simulink model "battery_model_closed_loop_simscape"  (R2016a)
settings: Solver=VariableStepAuto  StartTime=0.0  StopTime=6000  RelTol=1e-3
values from neighbouring files (symbols this model uses):
  C1 = tau1/R1    (= 240000)    [battery_and_controller_simscape_parameters.m]
  Cc = 1/(Q*wn*Rc)    [battery_and_controller_simscape_parameters.m]
  Ch = tauh/Rh    (= 40000)    [battery_and_controller_simscape_parameters.m]
  Cnom = 10    [battery_and_controller_simscape_parameters.m]
  Crate = 1.5*Mp*Cnom    (= 45)    [battery_and_controller_simscape_parameters.m]
  Gc0 = Gcwc*abs((1/wcp)*(i*wc)^2+(i*wc)+1)    [battery_and_controller_simscape_parameters.m]
  Lc = 1/(wn^2*Cc)    [battery_and_controller_simscape_parameters.m]
  Mp = 3    [battery_and_controller_simscape_parameters.m]
  Ns = 100    [battery_and_controller_simscape_parameters.m]
  R1 = 1e-3    (= 0.001)    [battery_and_controller_simscape_parameters.m]
  Rc = 5e3    (= 5000)    [battery_and_controller_simscape_parameters.m]
  Rs = Rp    (= 0.005)    [battery_and_controller_simscape_parameters.m]
  SOC_1 = 0.8    [battery_and_controller_simscape_parameters.m]
undefined symbols (not defined in the file or in its folder): V_soc
libraries: powerlib x49
settings Model: Creator=Gorkem  LastModifiedBy=Gorkem

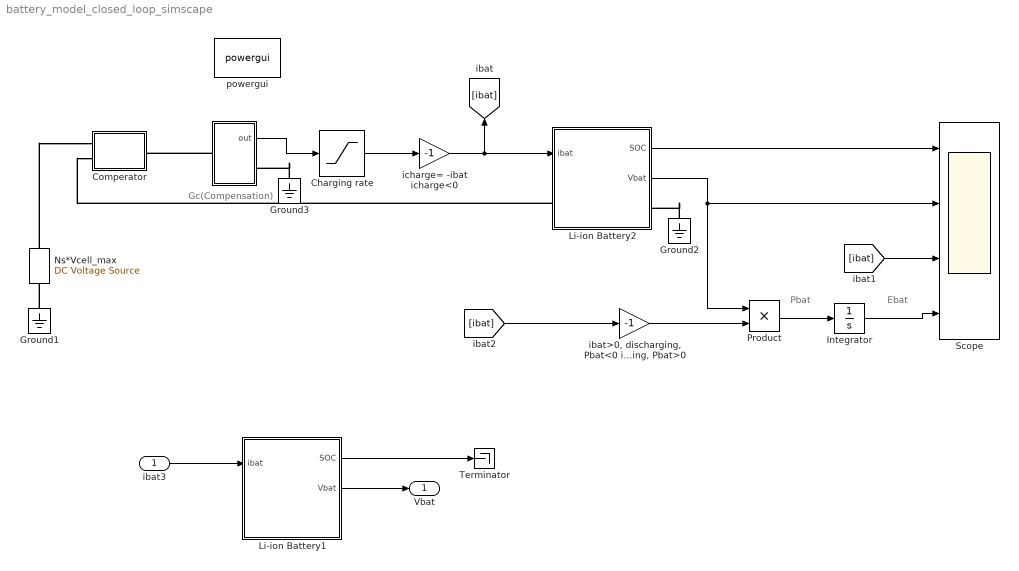
== system battery_model_closed_loop_simscape ==
  note: Gc(Compensation)
  note: Ebat
  note: Pbat
  ibat3 : Inport
  "  " : Subsystem
  Charging rate : Saturate  UpperLimit=Crate  LowerLimit=0
  Comperator : Subsystem
  Ground1 : powerlib/Elements/Ground  LConnTagsString=a
  Ground2 : powerlib/Elements/Ground  LConnTagsString=a
  Ground3 : powerlib/Elements/Ground  LConnTagsString=a
  Integrator : Integrator
  Li-ion Battery1 : Subsystem
  Li-ion Battery2 : Subsystem
  Ns*Vcell_max : powerlib/Electrical Sources/DC Voltage Source  Amplitude=3.7*Ns  Measurements=None
  Product : Product
  Scope : Scope  NumInputPorts=4
  Terminator : Terminator
  "ibat>0, discharging, Pbat<0 ibat<0, charging, Pbat>0" : Gain  Gain=-1
  icharge= -ibat icharge<0 : Gain  Gain=-1
  powergui : powerlib/powergui  Priority=1  SimulationMode=Continuous  SolverType=Tustin/Backward Euler (TBE)  SampleTime=50e-6  frequency=60  SPID=off  DisableSnubberDevices=off  DisableRonSwitches=off  DisableVfSwitches=off  SwTol=0  DisplayEquations=off  Interpol=off  ExternalGateDelay=off  methode=off  Ts=10  FunctionMessages=off  echomessages=off  HookPort=off  EnableUseOfTLC=off  x0status=blocks  frequencyindice=0  Pbase=100e6  ErrMax=1e-4  Iterations=50  UnitsV=kV  UnitsW=MW  buscounter=0  RestoreLinks=warning  ResistiveCurrentMeasurement=off  Frange=[0:2:500]  Ylog=off  Xlog=on  ShowGrid=off  save=off  variable=ZData  structure=0  ZoomFFT=off  StartTime=0.0  cycles=1  DisplayStyle=1  fundamental=60  FreqAxis=off  MaxFrequency=1000  frequencyindicesteady=1  RmsSteady=1  display=off
  Vbat : Outport
  wires:
  icharge= -ibat icharge<0/1 -> [ibat], Li-ion Battery2/1(ibat)
  Product/1 -> Integrator/1
  "ibat>0, discharging, Pbat<0 ibat<0, charging, Pbat>0"/1 -> Product/2
  Integrator/1 -> Scope/4
  Charging rate/1 -> icharge= -ibat icharge<0/1
  Li-ion Battery2/2(Vbat) -> Product/1, Scope/2
  Li-ion Battery2/1(SOC) -> Scope/1
  "  "/1("out ") -> Charging rate/1
  [ibat] -> "ibat>0, discharging, Pbat<0 ibat<0, charging, Pbat>0"/1
  [ibat] -> Scope/3
  ibat3/1 -> Li-ion Battery1/1(ibat)
  Li-ion Battery1/2(Vbat) -> Vbat/1
  Li-ion Battery1/1(SOC) -> Terminator/1
  connections:
  Ground1/LConn1 -- Ns*Vcell_max/LConn1
  Ground2/LConn1 -- Li-ion Battery2/RConn1
  Li-ion Battery2/LConn1 -- Comperator/LConn2
  Ns*Vcell_max/RConn1 -- Comperator/LConn1
  "  "/LConn1 -- Comperator/RConn1
  Ground3/LConn1 -- "  "/RConn1

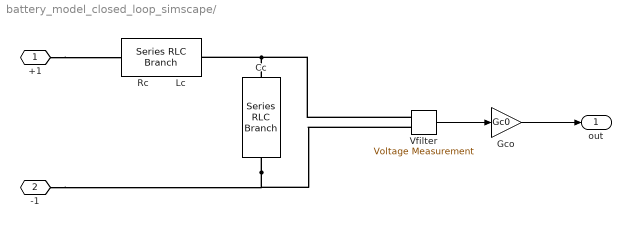
== system battery_model_closed_loop_simscape/   ==
  Cc : powerlib/Elements/Series RLC Branch  LConnTagsString=__new0  RConnTagsString=__new0  BranchType=C  Resistance=Rc  Inductance=Lc  SetiL0=off  InitialCurrent=0  Capacitance=Cc  Setx0=off  InitialVoltage=0  Measurements=None
  Gco : Gain  Gain=Gc0
  Rc         Lc : powerlib/Elements/Series RLC Branch  LConnTagsString=__new0  RConnTagsString=__new0  BranchType=RL  Resistance=Rc  Inductance=Lc  SetiL0=off  InitialCurrent=0  Capacitance=1e-6  Setx0=off  InitialVoltage=0  Measurements=None
  "Vfilter " : powerlib/Measurements/Voltage Measurement  PhasorSimulation=off  OutputType=Complex  PSBequivalent=0
  +1 : PMIOPort  Port=1  Side=Left
  -1 : PMIOPort  Port=2  Side=Right
  "out " : Outport
  wires:
  "Vfilter "/1 -> Gco/1
  Gco/1 -> "out "/1
  connections:
  +1/RConn1 -- Rc         Lc/LConn1
  Cc/LConn1 -- "Vfilter "/LConn1 -- Rc         Lc/RConn1
  Cc/RConn1 -- "Vfilter "/LConn2 -- -1/RConn1

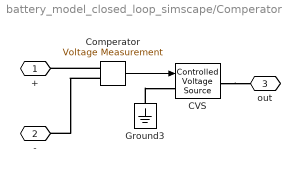
== system battery_model_closed_loop_simscape/Comperator ==
  CVS : powerlib/Electrical Sources/Controlled Voltage Source  Initialize=on  Source_Type=AC  Amplitude=0  Phase=0  Frequency=0  Measurements=None
  Comperator : powerlib/Measurements/Voltage Measurement  PhasorSimulation=off  OutputType=Complex  PSBequivalent=0
  Ground3 : powerlib/Elements/Ground  LConnTagsString=a
  + : PMIOPort  Port=1  Side=Left
  - : PMIOPort  Port=2  Side=Left
  out : PMIOPort  Port=3  Side=Right
  wires:
  Comperator/1 -> CVS/1
  connections:
  Ground3/LConn1 -- CVS/LConn1
  CVS/RConn1 -- out/RConn1
  Comperator/LConn2 -- -/RConn1
  Comperator/LConn1 -- +/RConn1

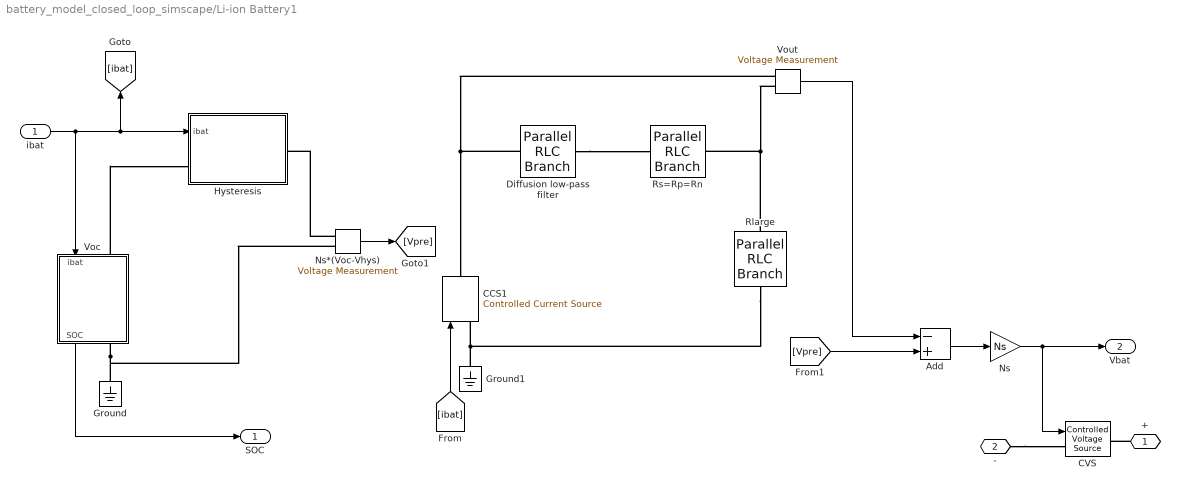
== system battery_model_closed_loop_simscape/Li-ion Battery1 ==
  ibat : Inport
  Add : Sum  Inputs=-+
  CCS1 : powerlib/Electrical Sources/Controlled Current Source  Initialize=off  Source_Type=AC  Amplitude=0  Phase=0  Frequency=0  Measurements=Current
  CVS : powerlib/Electrical Sources/Controlled Voltage Source  Initialize=on  Source_Type=AC  Amplitude=0  Phase=0  Frequency=0  Measurements=None
  Diffusion low-pass filter : powerlib/Elements/Parallel RLC Branch  LConnTagsString=a  RConnTagsString=__new0  BranchType=RC  Resistance=R1/Mp  Inductance=1e-3  SetiL0=off  InitialCurrent=0  Capacitance=C1*Mp  Setx0=off  InitialVoltage=0  Measurements=None
  Ground : powerlib/Elements/Ground  LConnTagsString=a
  Ground1 : powerlib/Elements/Ground  LConnTagsString=a
  Hysteresis : Subsystem
  Ns : Gain  Gain=Ns
  Ns*(Voc-Vhys) : powerlib/Measurements/Voltage Measurement  PhasorSimulation=off  OutputType=Complex  PSBequivalent=0
  Rlarge : powerlib/Elements/Parallel RLC Branch  LConnTagsString=a  RConnTagsString=__new0  BranchType=R  Resistance=1e15  Inductance=1e-3  SetiL0=off  InitialCurrent=0  Capacitance=C1*(Mp/Ns)  Setx0=off  InitialVoltage=0  Measurements=None
  Rs=Rp=Rn : powerlib/Elements/Parallel RLC Branch  LConnTagsString=a  RConnTagsString=__new0  BranchType=R  Resistance=Rs/Mp  Inductance=1e-3  SetiL0=off  InitialCurrent=0  Capacitance=C1*(Mp/Ns)  Setx0=off  InitialVoltage=0  Measurements=None
  Voc : Subsystem
  Vout : powerlib/Measurements/Voltage Measurement  PhasorSimulation=off  OutputType=Complex  PSBequivalent=0
  + : PMIOPort  Port=1  Side=Left
  - : PMIOPort  Port=2  Side=Right
  SOC : Outport
  Vbat : Outport  Port=2
  wires:
  Voc/1(SOC) -> SOC/1
  ibat/1 -> Voc/1(ibat), [ibat], Hysteresis/1(ibat)
  [ibat] -> CCS1/1
  Vout/1 -> Add/1
  Ns*(Voc-Vhys)/1 -> [Vpre]
  [Vpre] -> Add/2
  Add/1 -> Ns/1
  Ns/1 -> CVS/1, Vbat/1
  connections:
  Voc/LConn1 -- Hysteresis/LConn1
  Voc/RConn1 -- Ground/LConn1 -- Ns*(Voc-Vhys)/LConn2
  Diffusion low-pass filter/LConn1 -- Vout/LConn1 -- CCS1/RConn1
  Ground1/LConn1 -- CCS1/LConn1 -- Rlarge/RConn1
  Diffusion low-pass filter/RConn1 -- Rs=Rp=Rn/LConn1
  Vout/LConn2 -- Rlarge/LConn1 -- Rs=Rp=Rn/RConn1
  Ns*(Voc-Vhys)/LConn1 -- Hysteresis/RConn1
  +/RConn1 -- CVS/RConn1
  -/RConn1 -- CVS/LConn1

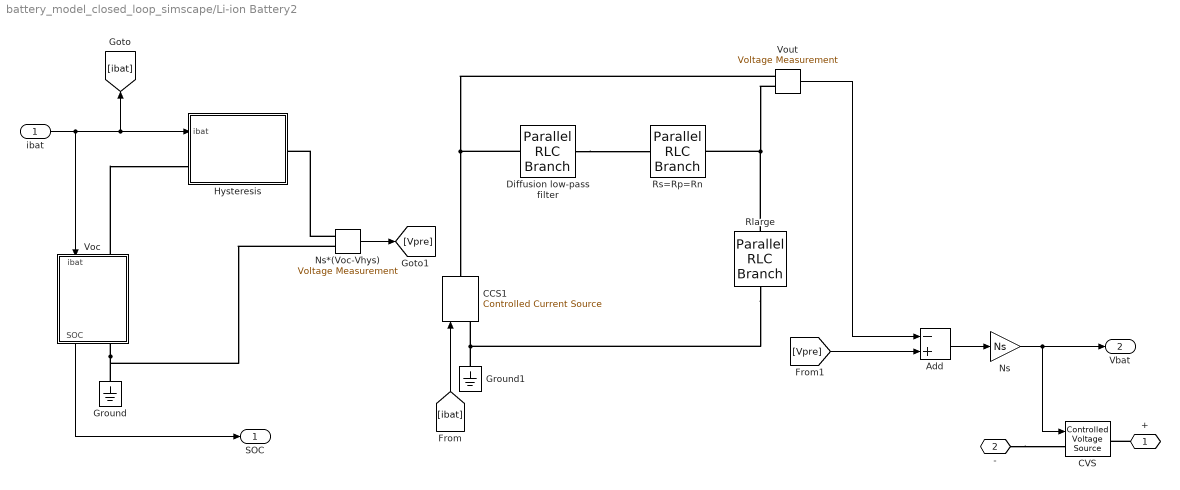
== system battery_model_closed_loop_simscape/Li-ion Battery2 ==
  ibat : Inport
  Add : Sum  Inputs=-+
  CCS1 : powerlib/Electrical Sources/Controlled Current Source  Initialize=off  Source_Type=AC  Amplitude=0  Phase=0  Frequency=0  Measurements=Current
  CVS : powerlib/Electrical Sources/Controlled Voltage Source  Initialize=on  Source_Type=AC  Amplitude=0  Phase=0  Frequency=0  Measurements=None
  Diffusion low-pass filter : powerlib/Elements/Parallel RLC Branch  LConnTagsString=a  RConnTagsString=__new0  BranchType=RC  Resistance=R1/Mp  Inductance=1e-3  SetiL0=off  InitialCurrent=0  Capacitance=C1*Mp  Setx0=off  InitialVoltage=0  Measurements=None
  Ground : powerlib/Elements/Ground  LConnTagsString=a
  Ground1 : powerlib/Elements/Ground  LConnTagsString=a
  Hysteresis : Subsystem
  Ns : Gain  Gain=Ns
  Ns*(Voc-Vhys) : powerlib/Measurements/Voltage Measurement  PhasorSimulation=off  OutputType=Complex  PSBequivalent=0
  Rlarge : powerlib/Elements/Parallel RLC Branch  LConnTagsString=a  RConnTagsString=__new0  BranchType=R  Resistance=1e15  Inductance=1e-3  SetiL0=off  InitialCurrent=0  Capacitance=C1*(Mp/Ns)  Setx0=off  InitialVoltage=0  Measurements=None
  Rs=Rp=Rn : powerlib/Elements/Parallel RLC Branch  LConnTagsString=a  RConnTagsString=__new0  BranchType=R  Resistance=Rs/Mp  Inductance=1e-3  SetiL0=off  InitialCurrent=0  Capacitance=C1*(Mp/Ns)  Setx0=off  InitialVoltage=0  Measurements=None
  Voc : Subsystem
  Vout : powerlib/Measurements/Voltage Measurement  PhasorSimulation=off  OutputType=Complex  PSBequivalent=0
  + : PMIOPort  Port=1  Side=Left
  - : PMIOPort  Port=2  Side=Right
  SOC : Outport
  Vbat : Outport  Port=2
  wires:
  Voc/1(SOC) -> SOC/1
  ibat/1 -> Voc/1(ibat), [ibat], Hysteresis/1(ibat)
  [ibat] -> CCS1/1
  Vout/1 -> Add/1
  Ns*(Voc-Vhys)/1 -> [Vpre]
  [Vpre] -> Add/2
  Add/1 -> Ns/1
  Ns/1 -> CVS/1, Vbat/1
  connections:
  Voc/LConn1 -- Hysteresis/LConn1
  Voc/RConn1 -- Ground/LConn1 -- Ns*(Voc-Vhys)/LConn2
  Diffusion low-pass filter/LConn1 -- Vout/LConn1 -- CCS1/RConn1
  Ground1/LConn1 -- CCS1/LConn1 -- Rlarge/RConn1
  Diffusion low-pass filter/RConn1 -- Rs=Rp=Rn/LConn1
  Vout/LConn2 -- Rlarge/LConn1 -- Rs=Rp=Rn/RConn1
  Ns*(Voc-Vhys)/LConn1 -- Hysteresis/RConn1
  +/RConn1 -- CVS/RConn1
  -/RConn1 -- CVS/LConn1

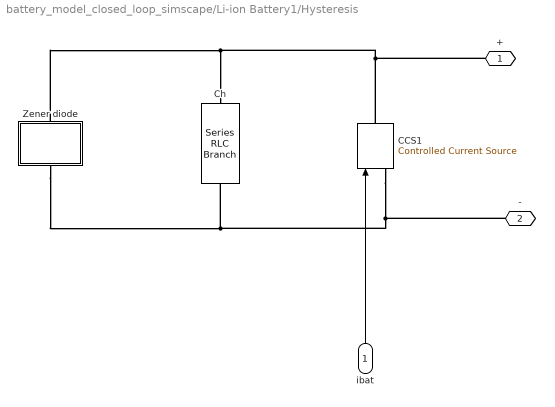
== system battery_model_closed_loop_simscape/Li-ion Battery1/Hysteresis ==
  ibat : Inport
  CCS1 : powerlib/Electrical Sources/Controlled Current Source  Initialize=off  Source_Type=AC  Amplitude=0  Phase=0  Frequency=0  Measurements=Current
  Ch : powerlib/Elements/Series RLC Branch  LConnTagsString=__new0  RConnTagsString=__new0  BranchType=C  Resistance=1  Inductance=1e-3  SetiL0=off  InitialCurrent=0  Capacitance=(Mp/Ns)*Ch  Setx0=off  InitialVoltage=0  Measurements=None
  Zener diode : Subsystem
  + : PMIOPort  Port=1  Side=Left
  - : PMIOPort  Port=2  Side=Right
  wires:
  ibat/1 -> CCS1/1
  connections:
  Zener diode/LConn1 -- Ch/LConn1 -- CCS1/RConn1 -- +/RConn1
  Zener diode/RConn1 -- Ch/RConn1 -- -/RConn1 -- CCS1/LConn1

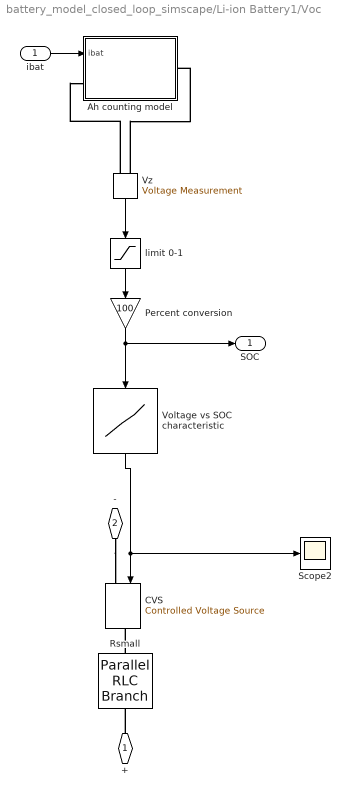
== system battery_model_closed_loop_simscape/Li-ion Battery1/Voc ==
  ibat : Inport
  Ah counting model : Subsystem
  CVS : powerlib/Electrical Sources/Controlled Voltage Source  Initialize=off  Source_Type=AC  Amplitude=0  Phase=0  Frequency=0  Measurements=Voltage
  Percent conversion : Gain  Gain=100
  Rsmall : powerlib/Elements/Parallel RLC Branch  LConnTagsString=a  RConnTagsString=__new0  BranchType=R  Resistance=1e-15  Inductance=1e-3  SetiL0=off  InitialCurrent=0  Capacitance=C1*(Mp/Ns)  Setx0=off  InitialVoltage=0  Measurements=None
  Scope2 : Scope
  Voltage vs SOC characteristic : Lookup_n-D  NumberOfTableDimensions=1  BreakpointsForDimension1=[0:9900]/100  Table=V_soc  InternalRulePriority=Speed  RndMeth=Simplest  InputSameDT=on
  Vz : powerlib/Measurements/Voltage Measurement  PhasorSimulation=off  OutputType=Complex  PSBequivalent=0
  limit 0-1 : Saturate  UpperLimit=SOC_1  LowerLimit=0
  + : PMIOPort  Port=1  Side=Left
  - : PMIOPort  Port=2  Side=Right
  SOC : Outport
  wires:
  Percent conversion/1 -> SOC/1, Voltage vs SOC characteristic/1
  Voltage vs SOC characteristic/1 -> Scope2/1, CVS/1
  Vz/1 -> limit 0-1/1
  limit 0-1/1 -> Percent conversion/1
  ibat/1 -> Ah counting model/1(ibat)
  connections:
  Vz/LConn2 -- Ah counting model/RConn1
  +/RConn1 -- Rsmall/RConn1
  Vz/LConn1 -- Ah counting model/LConn1
  -/RConn1 -- CVS/LConn1
  Rsmall/LConn1 -- CVS/RConn1

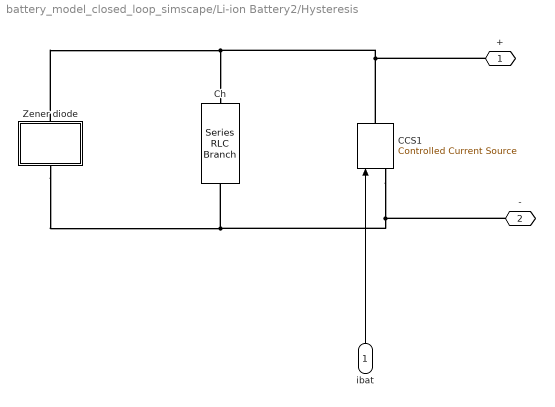
== system battery_model_closed_loop_simscape/Li-ion Battery2/Hysteresis ==
  ibat : Inport
  CCS1 : powerlib/Electrical Sources/Controlled Current Source  Initialize=off  Source_Type=AC  Amplitude=0  Phase=0  Frequency=0  Measurements=Current
  Ch : powerlib/Elements/Series RLC Branch  LConnTagsString=__new0  RConnTagsString=__new0  BranchType=C  Resistance=1  Inductance=1e-3  SetiL0=off  InitialCurrent=0  Capacitance=(Mp/Ns)*Ch  Setx0=off  InitialVoltage=0  Measurements=None
  Zener diode : Subsystem
  + : PMIOPort  Port=1  Side=Left
  - : PMIOPort  Port=2  Side=Right
  wires:
  ibat/1 -> CCS1/1
  connections:
  Zener diode/LConn1 -- Ch/LConn1 -- CCS1/RConn1 -- +/RConn1
  Zener diode/RConn1 -- Ch/RConn1 -- -/RConn1 -- CCS1/LConn1

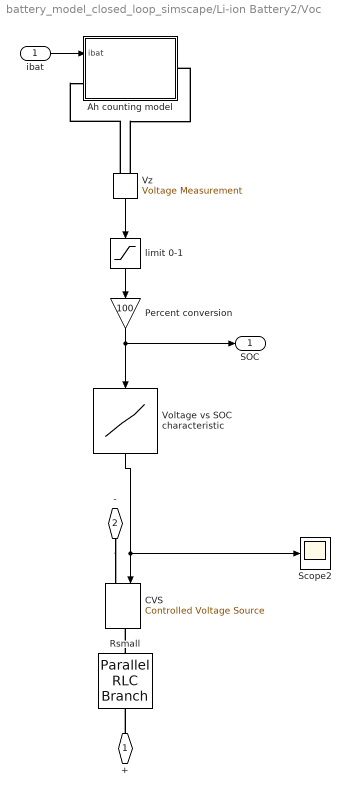
== system battery_model_closed_loop_simscape/Li-ion Battery2/Voc ==
  ibat : Inport
  Ah counting model : Subsystem
  CVS : powerlib/Electrical Sources/Controlled Voltage Source  Initialize=off  Source_Type=AC  Amplitude=0  Phase=0  Frequency=0  Measurements=Voltage
  Percent conversion : Gain  Gain=100
  Rsmall : powerlib/Elements/Parallel RLC Branch  LConnTagsString=a  RConnTagsString=__new0  BranchType=R  Resistance=1e-15  Inductance=1e-3  SetiL0=off  InitialCurrent=0  Capacitance=C1*(Mp/Ns)  Setx0=off  InitialVoltage=0  Measurements=None
  Scope2 : Scope
  Voltage vs SOC characteristic : Lookup_n-D  NumberOfTableDimensions=1  BreakpointsForDimension1=[0:9900]/100  Table=V_soc  InternalRulePriority=Speed  RndMeth=Simplest  InputSameDT=on
  Vz : powerlib/Measurements/Voltage Measurement  PhasorSimulation=off  OutputType=Complex  PSBequivalent=0
  limit 0-1 : Saturate  UpperLimit=SOC_1  LowerLimit=0
  + : PMIOPort  Port=1  Side=Left
  - : PMIOPort  Port=2  Side=Right
  SOC : Outport
  wires:
  Percent conversion/1 -> SOC/1, Voltage vs SOC characteristic/1
  Voltage vs SOC characteristic/1 -> Scope2/1, CVS/1
  Vz/1 -> limit 0-1/1
  limit 0-1/1 -> Percent conversion/1
  ibat/1 -> Ah counting model/1(ibat)
  connections:
  Vz/LConn2 -- Ah counting model/RConn1
  +/RConn1 -- Rsmall/RConn1
  Vz/LConn1 -- Ah counting model/LConn1
  -/RConn1 -- CVS/LConn1
  Rsmall/LConn1 -- CVS/RConn1

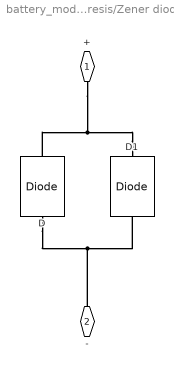
== system battery_model_closed_loop_simscape/Li-ion Battery1/Hysteresis/Zener diode ==
  D : powerlib/Power Electronics/Diode  Ron=0.001  Lon=0  Vf=Vm  IC=0  UseSnubber=off  Rs=inf  Cs=0  Measurements=off
  D1 : powerlib/Power Electronics/Diode  Ron=0.001  Lon=0  Vf=Vm  IC=0  UseSnubber=off  Rs=inf  Cs=0  Measurements=off
  + : PMIOPort  Port=1  Side=Left
  - : PMIOPort  Port=2  Side=Right
  connections:
  D1/LConn1 -- D/RConn1 -- +/RConn1
  D1/RConn1 -- D/LConn1 -- -/RConn1

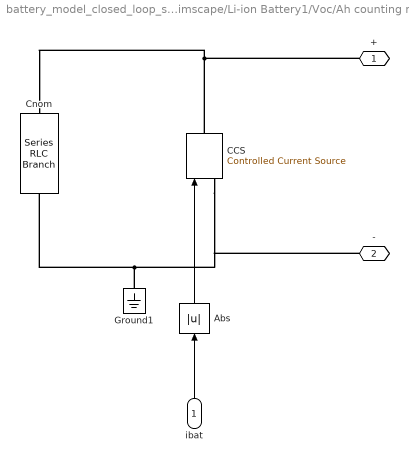
== system battery_model_closed_loop_simscape/Li-ion Battery1/Voc/Ah counting model ==
  ibat : Inport
  Abs : Abs
  CCS : powerlib/Electrical Sources/Controlled Current Source  Initialize=off  Source_Type=AC  Amplitude=0  Phase=0  Frequency=0  Measurements=Current
  Cnom : powerlib/Elements/Series RLC Branch  LConnTagsString=__new0  RConnTagsString=__new0  BranchType=C  Resistance=1  Inductance=1e-3  SetiL0=off  InitialCurrent=0  Capacitance=Cnom*Mp*3600  Setx0=on  InitialVoltage=SOC_0  Measurements=None
  Ground1 : powerlib/Elements/Ground  LConnTagsString=a
  + : PMIOPort  Port=1  Side=Left
  - : PMIOPort  Port=2  Side=Right
  wires:
  ibat/1 -> Abs/1
  Abs/1 -> CCS/1
  connections:
  CCS/RConn1 -- Cnom/LConn1 -- +/RConn1
  Ground1/LConn1 -- CCS/LConn1 -- -/RConn1 -- Cnom/RConn1

== system battery_model_closed_loop_simscape/Li-ion Battery2/Hysteresis/Zener diode ==
  D : powerlib/Power Electronics/Diode  Ron=0.001  Lon=0  Vf=Vm  IC=0  UseSnubber=off  Rs=inf  Cs=0  Measurements=off
  D1 : powerlib/Power Electronics/Diode  Ron=0.001  Lon=0  Vf=Vm  IC=0  UseSnubber=off  Rs=inf  Cs=0  Measurements=off
  + : PMIOPort  Port=1  Side=Left
  - : PMIOPort  Port=2  Side=Right
  connections:
  D1/LConn1 -- D/RConn1 -- +/RConn1
  D1/RConn1 -- D/LConn1 -- -/RConn1

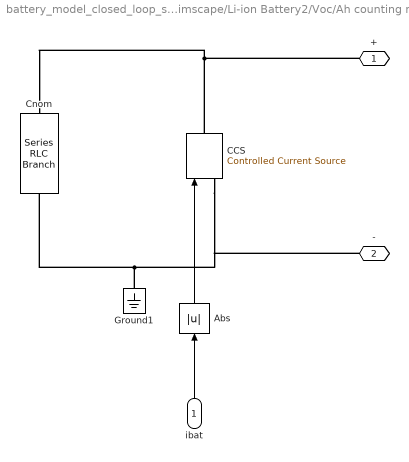
== system battery_model_closed_loop_simscape/Li-ion Battery2/Voc/Ah counting model ==
  ibat : Inport
  Abs : Abs
  CCS : powerlib/Electrical Sources/Controlled Current Source  Initialize=off  Source_Type=AC  Amplitude=0  Phase=0  Frequency=0  Measurements=Current
  Cnom : powerlib/Elements/Series RLC Branch  LConnTagsString=__new0  RConnTagsString=__new0  BranchType=C  Resistance=1  Inductance=1e-3  SetiL0=off  InitialCurrent=0  Capacitance=Cnom*Mp*3600  Setx0=on  InitialVoltage=SOC_0  Measurements=None
  Ground1 : powerlib/Elements/Ground  LConnTagsString=a
  + : PMIOPort  Port=1  Side=Left
  - : PMIOPort  Port=2  Side=Right
  wires:
  ibat/1 -> Abs/1
  Abs/1 -> CCS/1
  connections:
  CCS/RConn1 -- Cnom/LConn1 -- +/RConn1
  Ground1/LConn1 -- CCS/LConn1 -- -/RConn1 -- Cnom/RConn1
